simulink model "rectificador_pwm_plecs"  (R2024a)
settings: Solver=ode45  StartTime=0.0  StopTime=10  FixedStep=sim_sample_time  MaxStep=0.0001  RelTol=1e-3
undefined symbols (not defined in the file or in its folder): config, plecs
libraries: slpidlib x3
settings Model: SimulationMode=accelerator  PauseTimes=0.05  Creator=sebar  LastModifiedBy=sebar
settings SolverCC: AlgebraicLoopSolver=TrustRegion  AutoInsertRateTranBlk=on  DecoupledContinuousIntegration=on  ODENIntegrationMethod=ode14x
settings DataIOCC: ExternalInput=getinputstruct(op_trim1)  InitialState=steady_state  LimitDataPoints=on  SaveFinalState=on  SaveFormat=Structure  SaveOutput=off  SignalLogging=off  DSMLogging=off  SaveTime=off
settings OptimizationCC: LifeSpan=inf
settings DebuggingCC: ReadBeforeWriteMsg=DisableAll  WriteAfterWriteMsg=DisableAll  WriteAfterReadMsg=DisableAll  IgnoredZcDiagnostic=none  SolverPrmCheckMsg=warning  MultiTaskDSMMsg=none  SFUnexpectedBacktrackingDiag=warning  SFNoUnconditionalDefaultTransitionDiag=warning  SFExecutionAtInitializationDiag=none  ArithmeticOperatorsInVariantConditions=warning
settings HardwareCC: ProdBitPerPointer=32  ProdBitPerSizeT=32  ProdBitPerPtrDiffT=32  ProdLargestAtomicFloat=None  ProdIntDivRoundTo=Undefined  ProdEndianess=Unspecified  ProdWordSize=32  ProdHWDeviceType=32-bit Generic
settings ModelReferenceCC: UpdateModelReferenceTargets=IfOutOfDate  PropagateSignalLabelsOutOfModel=off
settings SFSimCC: SFSimEcho=off  SimUseLocalCustomCode=off  CustomCodeUndefinedFunction=UseInterfaceOnly  SimTargetLang=C++  GPUAcceleration=on  SimDLTargetLibrary=cudnn
settings RTWCC: RTWUseLocalCustomCode=off  GPUComputeCapability=3.5
settings CodeAppCC: StateflowObjectComments=on
settings GRTTargetCC: TargetLangStandard=C89/C90 (ANSI)
settings ConfigComp: CovMetricSettings=dw  CovSaveCumulativeToWorkspaceVar=on  CovSaveSingleToWorkspaceVar=on  CovExternalEMLEnable=off  CovSFcnEnable=off
settings SimscapeCC: SimscapeNormalizeSystem=off

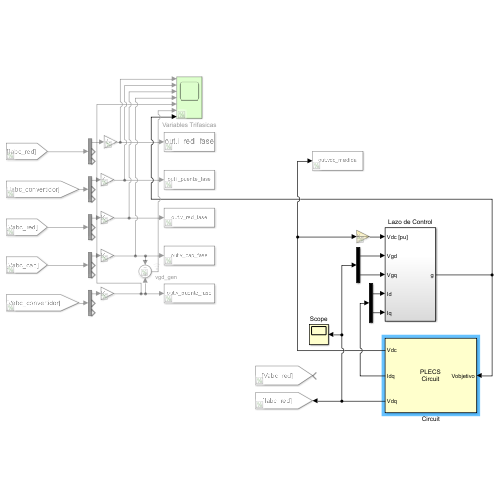
[thumbnail: Simulink's stored preview of the top-level diagram]
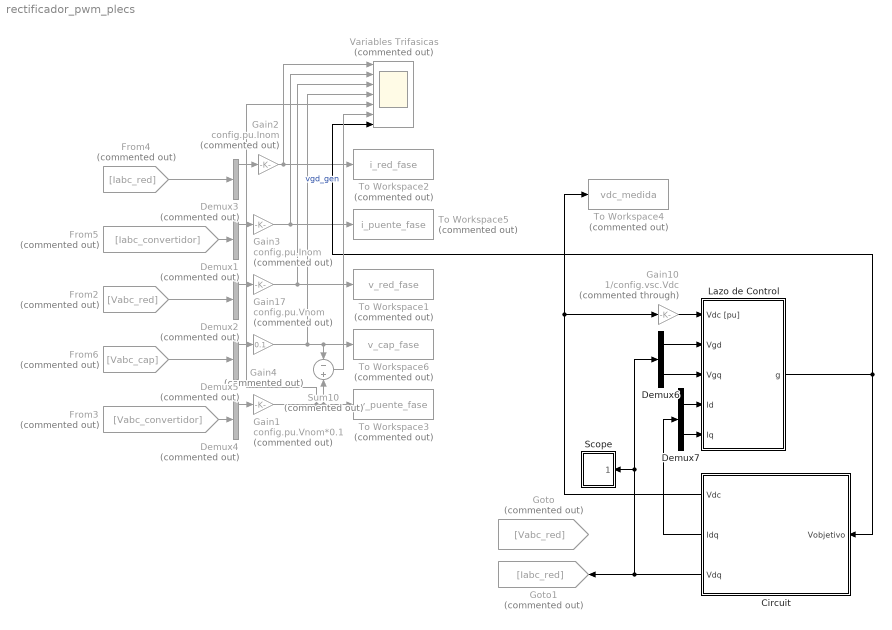
== system rectificador_pwm_plecs ==
  Circuit : Subsystem  LoadFcn=plecs('sl', 200);  InitFcn=plecs('sl', 214);  StartFcn=plecs('sl', 208);  StopFcn=plecs('sl', 209);  mask(PlecsCircuit){PLECSData=<binary blob, 10204 chars, not shown>}
      mask prompts: PLECSData "PLECS Data (Do not delete or modify!)"
      mask init:
      | % PLACE CUSTOM INITIALIZATIONS ABOVE
      | % DO NOT REMOVE
      | plecs('sl', 215);
      | % DO NOT REMOVE
      settings: CopyFcn=plecs('sl', 203);  DeleteFcn=plecs('sl', 205);  UndoDeleteFcn=plecs('sl', 206);  PreSaveFcn=plecs('sl', 211);  PostSaveFcn=plecs('sl', 201);  NameChangeFcn=plecs('sl', 210);  DestroyFcn=plecs('sl', 207);  PreCopyFcn=plecs('sl', 216);  OpenFcn=plecs('sl', 202);  ErrorFcn=plerrorfcn
      mask Help: eval('plecs(''help'', ''qthelp:///creatingacircuit.html'')')
      mask Display: disp('PLECS\nCircuit')
  Demux{1..5} (5 alike) : Demux  Commented=on  Outputs=3
  Demux6 : Demux  Outputs=2
  Demux7 : Demux  Outputs=2
  From2 : From  Commented=on  GotoTag=Vabc_red
  From3 : From  Commented=on  GotoTag=Vabc_convertidor
  From4 : From  Commented=on  GotoTag=Iabc_red
  From5 : From  Commented=on  GotoTag=Iabc_convertidor
  From6 : From  Commented=on  GotoTag=Vabc_cap
  Gain1 : Gain  Commented=on  Gain=config.pu.Vnom*0.1
  Gain10 : Gain  Commented=through  Gain=1/config.vsc.Vdc
  Gain17 : Gain  Commented=on  Gain=config.pu.Vnom
  Gain2 : Gain  Commented=on  Gain=config.pu.Inom
  Gain3 : Gain  Commented=on  Gain=config.pu.Inom
  Gain4 : Gain  Commented=on  Gain=0.1
  Goto : Goto  Commented=on  GotoTag=Vabc_red
  Goto1 : Goto  Commented=on  GotoTag=Iabc_red
  Lazo de Control : Subsystem
  Scope : Subsystem  LoadFcn=plecs('sl', 300);  InitFcn=plecs('sl', 314);  StartFcn=plecs('sl', 308);  StopFcn=plecs('sl', 309);  mask{Settings=<binary blob, 728 chars, not shown>}
      mask init:
      | plecs('sl', 315);
      settings: CopyFcn=plecs('sl', 303);  DeleteFcn=plecs('sl', 305);  UndoDeleteFcn=plecs('sl', 306);  PreSaveFcn=plecs('sl', 311);  NameChangeFcn=plecs('sl', 310);  DestroyFcn=plecs('sl', 307);  OpenFcn=plecs('sl', 302);  ErrorFcn=plerrorfcn
      mask Display: plot([0.1 0.9 0.9 0.1 0.1], [0.9 0.9 0.5 0.5 0.9])
  Sum10 : Sum  Commented=on  Inputs=-|+
  To Workspace1 : ToWorkspace  Commented=on  VariableName=v_red_fase  SaveFormat=Timeseries  SampleTime=config.to_workspace_sample_time
  To Workspace2 : ToWorkspace  Commented=on  VariableName=i_red_fase  SaveFormat=Timeseries  SampleTime=config.to_workspace_sample_time
  To Workspace3 : ToWorkspace  Commented=on  VariableName=v_puente_fase  SaveFormat=Timeseries  SampleTime=config.to_workspace_sample_time
  To Workspace4 : ToWorkspace  Commented=on  VariableName=vdc_medida  SaveFormat=Timeseries  SampleTime=config.to_workspace_sample_time
  To Workspace5 : ToWorkspace  Commented=on  VariableName=i_puente_fase  SaveFormat=Timeseries  SampleTime=config.to_workspace_sample_time
  To Workspace6 : ToWorkspace  Commented=on  VariableName=v_cap_fase  SaveFormat=Timeseries  SampleTime=config.to_workspace_sample_time
  Variables Trifasicas : Scope  Commented=on  NumInputPorts=7
  wires:
  Gain10/1 -> Lazo de Control/1(Vdc [pu])
  Circuit/1(Vdc) -> To Workspace4/1, Gain10/1
  Gain17/1 -> To Workspace1/1, Variables Trifasicas/3
  Gain1/1 -> Sum10/2, To Workspace3/1, Variables Trifasicas/5
  Gain2/1 -> Variables Trifasicas/1, To Workspace2/1
  Gain3/1 -> Variables Trifasicas/2, To Workspace5/1
  Lazo de Control/1(g) -> Circuit/1(Vobjetivo), Variables Trifasicas/7
  From4/1 -> Demux3/1
  Demux3/1 -> Gain2/1
  Demux1/1 -> Gain3/1
  Demux2/1 -> Gain17/1
  Demux4/1 -> Gain1/1
  From3/1 -> Demux4/1
  From2/1 -> Demux2/1
  From5/1 -> Demux1/1
  From6/1 -> Demux5/1
  Gain4/1 -> Sum10/1, To Workspace6/1, Variables Trifasicas/4
  Demux5/1 -> Gain4/1
  Sum10/1 -> Variables Trifasicas/6  "vgd_gen"
  Circuit/3(Vdq) -> Goto1/1, Demux6/1, Scope/1(1)
  Demux6/1 -> Lazo de Control/2(Vgd)
  Demux6/2 -> Lazo de Control/3(Vgq)
  Circuit/2(Idq) -> Demux7/1
  Demux7/1 -> Lazo de Control/4(Id)
  Demux7/2 -> Lazo de Control/5(Iq)

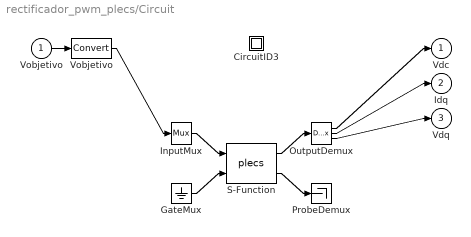
== system rectificador_pwm_plecs/Circuit ==
  Vobjetivo : Inport  PortDimensions=2
  " CircuitID3 " : Subsystem
  " GateMux " : Ground
  " InputMux " : Mux  Inputs=[ 2 ]
  " OutputDemux " : Demux  Outputs=[ 1 2 2 ]
  " ProbeDemux " : Terminator
  " S-Function " : S-Function  FunctionName=plecs  SFunctionDeploymentMode=off  EnableBusSupport=off
  " Vobjetivo " : DataTypeConversion
  Vdc : Outport  PortDimensions=1
  Idq : Outport  Port=2  PortDimensions=2
  Vdq : Outport  Port=3  PortDimensions=2
  wires:
  " InputMux "/1 -> " S-Function "/1
  " GateMux "/1 -> " S-Function "/2
  " S-Function "/1 -> " OutputDemux "/1
  " S-Function "/2 -> " ProbeDemux "/1
  Vobjetivo/1 -> " Vobjetivo "/1
  " Vobjetivo "/1 -> " InputMux "/1
  " OutputDemux "/1 -> Vdc/1
  " OutputDemux "/2 -> Idq/1
  " OutputDemux "/3 -> Vdq/1

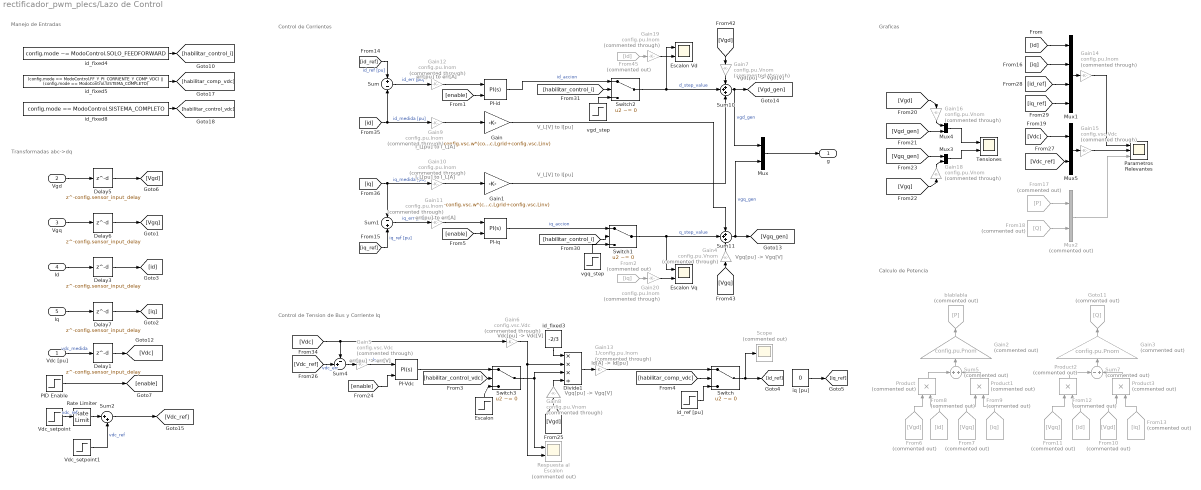
== system rectificador_pwm_plecs/Lazo de Control ==
  note: Transformadas abc->dq
  note: I_L[pu] to I_L[A]
  note: Calculo de Potencia
  note: Graficas
  note: Manejo de Entradas
  note: Control de Tension de Bus y Corriente Iq
  note: Control de Corrientes
  note: V_L[V] to I[pu]
  note: Vgd[pu] -> Vgd[V]
  note: I_L[pu] to I_L[A]
  note: Vgq[pu] -> Vgq[V]
  note: Vgq[pu] -> Vgq[V]
  note: Id[A] -> Id[pu]
  note: err[pu] -> err[V]
  note: err[pu] to err[A]
  note: err[pu] to err[A]
  note: Vdc[pu] -> Vdc[V]
  note: V_L[V] to I[pu]
  Vdc [pu] : Inport
  Vgd : Inport  Port=2
  Vgq : Inport  Port=3
  Id : Inport  Port=4
  Iq : Inport  Port=5
  Delay{1,3,5..7} (5 alike) : Delay  DelayLength=config.sensor_input_delay  InitialCondition=1  SampleTime=config.sensor_input_sample_time
  Divide1 : Product  Inputs=***/
  Escalon : Step  Time=config.step.id.time  Before=config.step.id.start_value  After=config.step.id.end_value  SampleTime=1e-5
  Escalon Vd : Scope  NumInputPorts=2
  Escalon Vq : Scope  NumInputPorts=2
  From10 : From  Commented=on  GotoTag=Vgd
  From11 : From  Commented=on  GotoTag=Vgq
  From12 : From  Commented=on  GotoTag=id
  From13 : From  Commented=on  GotoTag=iq
  From17 : From  Commented=on  GotoTag=P
  From18 : From  Commented=on  GotoTag=Q
  From2 : From  Commented=on  GotoTag=iq
  From45 : From  Commented=on  GotoTag=id
  From6 : From  Commented=on  GotoTag=Vgd
  From7 : From  Commented=on  GotoTag=Vgq
  From8 : From  Commented=on  GotoTag=id
  From9 : From  Commented=on  GotoTag=iq
  Gain : Gain  Gain=config.vsc.w*(config.vsc.Lgrid+config.vsc.Linv)
  Gain1 : Gain  Gain=-config.vsc.w*(config.vsc.Lgrid+config.vsc.Linv)
  Gain{9..12,14,19..20} (7 alike) : Gain  Commented=through  Gain=config.pu.Inom
  Gain13 : Gain  Commented=through  Gain=1/config.pu.Inom
  Gain15 : Gain  Commented=through  Gain=config.vsc.Vdc
  Gain{4,7..8,16,18} (5 alike) : Gain  Commented=through  Gain=config.pu.Vnom
  Gain2 : Gain  Commented=on  Gain=config.pu.Pnom
  Gain3 : Gain  Commented=on  Gain=config.pu.Pnom
  Gain5 : Gain  Commented=through  Gain=config.vsc.Vdc
  Gain6 : Gain  Commented=through  Gain=config.vsc.Vdc
  Goto11 : Goto  Commented=on  GotoTag=Q
  Mux{,3..5} (4 alike) : Mux  Inputs=2
  Mux1 : Mux
  Mux2 : Mux  Commented=on  Inputs=2
  PI-Vdc : slpidlib/PID Controller  Controller=PI  Form=Parallel  TimeDomain=Continuous-time  UseExternalTs=off  SampleTime=1  IntegratorMethod=Forward Euler  FilterMethod=Forward Euler  ControllerParametersSource=internal  P=config.ContDC.Kp  I=config.ContDC.Ki  UseKiTs=off  D=0  UseExternalDerivativeSource=off  N=100  UseFilter=on  TunerSelectOption=Transfer Function Based (PID Tuner App)  InitialConditionSource=internal  InitialConditionForIntegrator=12.92  InitialConditionForFilter=0  DifferentiatorICPrevScaledInput=0  ExternalReset=level  TrackingMode=off  Kt=1  LimitOutput=off  SatLimitsSource=internal  UpperSaturationLimit=inf  LowerSaturationLimit=-inf  LinearizeAsGain=on  AntiWindupMode=none  Kb=1  LimitIntegrator=off  UpperIntegratorSaturationLimit=inf  LowerIntegratorSaturationLimit=-inf  POutMin=[]  POutMax=[]  IOutMin=[]  IOutMax=[]  DOutMin=[]  DOutMax=[]  NOutMin=[]  NOutMax=[]  SumOutMin=[]  SumOutMax=[]  SaturationOutMin=[]  SaturationOutMax=[]  PParamMin=[]  PParamMax=[]  IParamMin=[]  IParamMax=[]  DParamMin=[]  DParamMax=[]  NParamMin=[]  NParamMax=[]  KbParamMin=[]  KbParamMax=[]  KtParamMin=[]  KtParamMax=[]  KbOutMin=[]  KbOutMax=[]  KtOutMin=[]  KtOutMax=[]  IntegratorOutMin=[]  IntegratorOutMax=[]  FilterOutMin=[]  FilterOutMax=[]  SumI1OutMin=[]  SumI1OutMax=[]  SumI2OutMin=[]  SumI2OutMax=[]  SumI3OutMin=[]  SumI3OutMax=[]  SumI4OutMin=[]  SumI4OutMax=[]  SumDOutMin=[]  SumDOutMax=[]  DifferentiatorOutMin=[]  DifferentiatorOutMax=[]  FilterDiffOutCoefMin=[]  FilterDiffOutCoefMax=[]  ReciprocalOutMin=[]  ReciprocalOutMax=[]  SumDenOutMin=[]  SumDenOutMax=[]  SumNumOutMin=[]  SumNumOutMax=[]  DivideOutMin=[]  DivideOutMax=[]  UdiffTsProdOutMin=[]  UdiffTsProdOutMax=[]  NTsProdOutMin=[]  NTsProdOutMax=[]  UintegralTsProdOutMin=[]  UintegralTsProdOutMax=[]  UngainTsProdOutMin=[]  UngainTsProdOutMax=[]  ClampingZeroOutDataTypeStr=Inherit: Inherit via back propagation  ClampingZeroOutMin=[]  ClampingZeroOutMax=[]  FilterDenConstantOutDataTypeStr=Inherit: Inherit via back propagation  FilterDenConstantOutMin=[]  FilterDenConstantOutMax=[]  PCopyOutDataTypeStr=Inherit: Inherit via back propagation  PCopyOutMin=[]  PCopyOutMax=[]  NCopyOutDataTypeStr=Inherit: Inherit via back propagation  NCopyOutMin=[]  NCopyOutMax=[]  IntegratorContinuousStateAttributes=''  IntegratorStateMustResolveToSignalObject=off  IntegratorRTWStateStorageClass=Auto  FilterContinuousStateAttributes=''  FilterStateMustResolveToSignalObject=off  FilterRTWStateStorageClass=Auto  ParallelPVariant=InternalParameters  IdealPVariant=Disabled  IVariant=InternalParameters  DVariant=Disabled  IntegratorVariant=Continuous  SatVariant=Disabled  AWVariant=Passthrough  PCopyVariant=Disabled  TRVariant=Disabled  FdbkBlocksVariant=Forward  IdealPFdbkVariant=Disabled  SatFdbkVariant=Disabled  DerivativeFilterVariant=Disabled  NVariant=Disabled  NCopyVariant=Disabled_SignalSpec  FilterICVariant=Disabled  IntegratorICVariant=InternalICs  ExternalResetVariant=ExternalReset  TRSumVariant=Passthrough  SumFdbkVariant=Disabled  SumVariant=Sum_PI  TsampFilterVariant=InternalTs  TsampNgainVariant=Passthrough  TsampIntegralVariant=Disabled_SignalSpec  ExternalSaturationOutDataTypeStr=Inherit: Same as second input  DerivativeSourceVariant=Disabled
  PI-id : slpidlib/PID Controller  Controller=PI  Form=Parallel  TimeDomain=Continuous-time  UseExternalTs=off  SampleTime=1  IntegratorMethod=Forward Euler  FilterMethod=Forward Euler  ControllerParametersSource=internal  P=config.ContI.Kp  I=config.ContI.Ki  UseKiTs=off  D=0  UseExternalDerivativeSource=off  N=100  UseFilter=on  TunerSelectOption=Transfer Function Based (PID Tuner App)  InitialConditionSource=internal  InitialConditionForIntegrator=-1.85  InitialConditionForFilter=0  DifferentiatorICPrevScaledInput=0  ExternalReset=level  TrackingMode=off  Kt=1  LimitOutput=off  SatLimitsSource=internal  UpperSaturationLimit=-4  LowerSaturationLimit=-20  LinearizeAsGain=on  AntiWindupMode=clamping  Kb=1  LimitIntegrator=off  UpperIntegratorSaturationLimit=inf  LowerIntegratorSaturationLimit=-inf  POutMin=[]  POutMax=[]  IOutMin=[]  IOutMax=[]  DOutMin=[]  DOutMax=[]  NOutMin=[]  NOutMax=[]  SumOutMin=[]  SumOutMax=[]  SaturationOutMin=[]  SaturationOutMax=[]  PParamMin=[]  PParamMax=[]  IParamMin=[]  IParamMax=[]  DParamMin=[]  DParamMax=[]  NParamMin=[]  NParamMax=[]  KbParamMin=[]  KbParamMax=[]  KtParamMin=[]  KtParamMax=[]  KbOutMin=[]  KbOutMax=[]  KtOutMin=[]  KtOutMax=[]  IntegratorOutMin=[]  IntegratorOutMax=[]  FilterOutMin=[]  FilterOutMax=[]  SumI1OutMin=[]  SumI1OutMax=[]  SumI2OutMin=[]  SumI2OutMax=[]  SumI3OutMin=[]  SumI3OutMax=[]  SumI4OutMin=[]  SumI4OutMax=[]  SumDOutMin=[]  SumDOutMax=[]  DifferentiatorOutMin=[]  DifferentiatorOutMax=[]  FilterDiffOutCoefMin=[]  FilterDiffOutCoefMax=[]  ReciprocalOutMin=[]  ReciprocalOutMax=[]  SumDenOutMin=[]  SumDenOutMax=[]  SumNumOutMin=[]  SumNumOutMax=[]  DivideOutMin=[]  DivideOutMax=[]  UdiffTsProdOutMin=[]  UdiffTsProdOutMax=[]  NTsProdOutMin=[]  NTsProdOutMax=[]  UintegralTsProdOutMin=[]  UintegralTsProdOutMax=[]  UngainTsProdOutMin=[]  UngainTsProdOutMax=[]  ClampingZeroOutDataTypeStr=Inherit: Inherit via back propagation  ClampingZeroOutMin=[]  ClampingZeroOutMax=[]  FilterDenConstantOutDataTypeStr=Inherit: Inherit via back propagation  FilterDenConstantOutMin=[]  FilterDenConstantOutMax=[]  PCopyOutDataTypeStr=Inherit: Inherit via back propagation  PCopyOutMin=[]  PCopyOutMax=[]  NCopyOutDataTypeStr=Inherit: Inherit via back propagation  NCopyOutMin=[]  NCopyOutMax=[]  IntegratorContinuousStateAttributes=''  IntegratorStateMustResolveToSignalObject=off  IntegratorRTWStateStorageClass=Auto  FilterContinuousStateAttributes=''  FilterStateMustResolveToSignalObject=off  FilterRTWStateStorageClass=Auto  ParallelPVariant=InternalParameters  IdealPVariant=Disabled  IVariant=InternalParameters  DVariant=Disabled  IntegratorVariant=Continuous  SatVariant=Disabled  AWVariant=Passthrough  PCopyVariant=Disabled  TRVariant=Disabled  FdbkBlocksVariant=Forward  IdealPFdbkVariant=Disabled  SatFdbkVariant=Disabled  DerivativeFilterVariant=Disabled  NVariant=Disabled  NCopyVariant=Disabled_SignalSpec  FilterICVariant=Disabled  IntegratorICVariant=InternalICs  ExternalResetVariant=ExternalReset  TRSumVariant=Passthrough  SumFdbkVariant=Disabled  SumVariant=Sum_PI  TsampFilterVariant=InternalTs  TsampNgainVariant=Passthrough  TsampIntegralVariant=Disabled_SignalSpec  ExternalSaturationOutDataTypeStr=Inherit: Same as second input  DerivativeSourceVariant=Disabled
  PI-iq : slpidlib/PID Controller  Controller=PI  Form=Parallel  TimeDomain=Continuous-time  UseExternalTs=off  SampleTime=1  IntegratorMethod=Forward Euler  FilterMethod=Forward Euler  ControllerParametersSource=internal  P=config.ContI.Kp  I=config.ContI.Ki  UseKiTs=off  D=0  UseExternalDerivativeSource=off  N=100  UseFilter=on  TunerSelectOption=Transfer Function Based (PID Tuner App)  InitialConditionSource=internal  InitialConditionForIntegrator=0  InitialConditionForFilter=0  DifferentiatorICPrevScaledInput=0  ExternalReset=level  TrackingMode=off  Kt=1  LimitOutput=off  SatLimitsSource=internal  UpperSaturationLimit=20  LowerSaturationLimit=-20  LinearizeAsGain=on  AntiWindupMode=none  Kb=1  LimitIntegrator=off  UpperIntegratorSaturationLimit=inf  LowerIntegratorSaturationLimit=-inf  POutMin=[]  POutMax=[]  IOutMin=[]  IOutMax=[]  DOutMin=[]  DOutMax=[]  NOutMin=[]  NOutMax=[]  SumOutMin=[]  SumOutMax=[]  SaturationOutMin=[]  SaturationOutMax=[]  PParamMin=[]  PParamMax=[]  IParamMin=[]  IParamMax=[]  DParamMin=[]  DParamMax=[]  NParamMin=[]  NParamMax=[]  KbParamMin=[]  KbParamMax=[]  KtParamMin=[]  KtParamMax=[]  KbOutMin=[]  KbOutMax=[]  KtOutMin=[]  KtOutMax=[]  IntegratorOutMin=[]  IntegratorOutMax=[]  FilterOutMin=[]  FilterOutMax=[]  SumI1OutMin=[]  SumI1OutMax=[]  SumI2OutMin=[]  SumI2OutMax=[]  SumI3OutMin=[]  SumI3OutMax=[]  SumI4OutMin=[]  SumI4OutMax=[]  SumDOutMin=[]  SumDOutMax=[]  DifferentiatorOutMin=[]  DifferentiatorOutMax=[]  FilterDiffOutCoefMin=[]  FilterDiffOutCoefMax=[]  ReciprocalOutMin=[]  ReciprocalOutMax=[]  SumDenOutMin=[]  SumDenOutMax=[]  SumNumOutMin=[]  SumNumOutMax=[]  DivideOutMin=[]  DivideOutMax=[]  UdiffTsProdOutMin=[]  UdiffTsProdOutMax=[]  NTsProdOutMin=[]  NTsProdOutMax=[]  UintegralTsProdOutMin=[]  UintegralTsProdOutMax=[]  UngainTsProdOutMin=[]  UngainTsProdOutMax=[]  ClampingZeroOutDataTypeStr=Inherit: Inherit via back propagation  ClampingZeroOutMin=[]  ClampingZeroOutMax=[]  FilterDenConstantOutDataTypeStr=Inherit: Inherit via back propagation  FilterDenConstantOutMin=[]  FilterDenConstantOutMax=[]  PCopyOutDataTypeStr=Inherit: Inherit via back propagation  PCopyOutMin=[]  PCopyOutMax=[]  NCopyOutDataTypeStr=Inherit: Inherit via back propagation  NCopyOutMin=[]  NCopyOutMax=[]  IntegratorContinuousStateAttributes=''  IntegratorStateMustResolveToSignalObject=off  IntegratorRTWStateStorageClass=Auto  FilterContinuousStateAttributes=''  FilterStateMustResolveToSignalObject=off  FilterRTWStateStorageClass=Auto  ParallelPVariant=InternalParameters  IdealPVariant=Disabled  IVariant=InternalParameters  DVariant=Disabled  IntegratorVariant=Continuous  SatVariant=Disabled  AWVariant=Passthrough  PCopyVariant=Disabled  TRVariant=Disabled  FdbkBlocksVariant=Forward  IdealPFdbkVariant=Disabled  SatFdbkVariant=Disabled  DerivativeFilterVariant=Disabled  NVariant=Disabled  NCopyVariant=Disabled_SignalSpec  FilterICVariant=Disabled  IntegratorICVariant=InternalICs  ExternalResetVariant=ExternalReset  TRSumVariant=Passthrough  SumFdbkVariant=Disabled  SumVariant=Sum_PI  TsampFilterVariant=InternalTs  TsampNgainVariant=Passthrough  TsampIntegralVariant=Disabled_SignalSpec  ExternalSaturationOutDataTypeStr=Inherit: Same as second input  DerivativeSourceVariant=Disabled
  PID Enable : Step  Time=1.5  Before=1  After=0  SampleTime=1e-5
  Parametros Relevantes : Scope  NumInputPorts=3
  Product{,1..3} (4 alike) : Product  Commented=on
  Rate Limiter : RateLimiter  RisingSlewLimit=15  SampleTimeMode=inherited
  Respuesta al Escalon : Scope  Commented=on  NumInputPorts=2
  Scope : Scope  Commented=on
  Sum : Sum  Inputs=+|-
  Sum1 : Sum  Inputs=-|+
  Sum10 : Sum  Inputs=+++
  Sum11 : Sum  Inputs=+++
  Sum2 : Sum  Inputs=|++
  Sum4 : Sum  Inputs=-+|
  Sum5 : Sum  Commented=on  Inputs=+|+
  Sum7 : Sum  Commented=on  Inputs=-|+
  Switch{,1..3} (4 alike) : Switch  Criteria=u2 ~= 0  SaturateOnIntegerOverflow=off  InputSameDT=off
  Tensiones : Scope  NumInputPorts=2
  Vdc_setpoint : Step  Time=1.5  Before=config.vsc.Vgrid*sqrt(2)*3*sqrt(3)/pi*0+350  After=config.vsc.Vdc*0+350  SampleTime=0
  Vdc_setpoint1 : Step  Time=7  After=50  SampleTime=0
  blablabla : Goto  Commented=on  GotoTag=P
  id_fixed3 : Constant  Value=-2/3
  id_fixed4 : Constant  Value=config.mode ~= ModoControl.SOLO_FEEDFORWARD
  id_fixed5 : Constant  Value=(config.mode == ModoControl.FF_Y_PI_CORRIENTE_Y_COMP_VDC) || (config.mode == ModoControl.SISTEMA_COMPLETO)
  id_fixed8 : Constant  Value=config.mode == ModoControl.SISTEMA_COMPLETO
  id_ref [pu] : Step  Time=1.25  Before=-3.0707/config.pu.Inom  After=-3.0707/config.pu.Inom*(1 + config.step_setpoint_corriente/100)  SampleTime=0
  iq [pu] : Constant  Value=0
  vgd_step : Step  Time=config.step.vgd.time  Before=config.step.vgd.start_value  After=config.step.vgd.end_value  SampleTime=1e-5
  vgq_step : Step  Time=config.step.vgq.time  Before=config.step.vgq.start_value  After=config.step.vgq.end_value  SampleTime=1e-5
  g : Outport
  wires:
  Vgq/1 -> Delay6/1
  [id] -> Gain9/1, Sum/2  "id_medida [pu]"
  [iq] -> Gain10/1, Sum1/1  "iq_medida [pu]"
  [id_ref] -> Sum/1  "id_ref [pu]"
  [iq_ref] -> Sum1/2  "iq_ref [pu]"
  Sum/1 -> Gain12/1  "id_err [pu]"
  Sum1/1 -> Gain11/1  "iq_err [pu]"
  PI-iq/1 -> Switch1/1  "iq_accion"
  Sum11/1 -> Mux/2, [Vgq_gen]  "vgq_gen"
  Vdc [pu]/1 -> Delay1/1  "vdc_medida"
  Gain5/1 -> PI-Vdc/1  "vdc_err"
  Divide1/1 -> Gain13/1
  id_ref [pu]/1 -> Switch/3
  iq [pu]/1 -> [iq_ref]
  From17/1 -> Mux2/1
  From18/1 -> Mux2/2
  [iq] -> Mux1/2
  [id] -> Mux1/1
  [Vdc] -> Mux5/1
  Mux1/1 -> Gain14/1
  Mux2/1 -> Parametros Relevantes/3
  [Vgd_gen] -> Mux4/2
  [Vgq_gen] -> Mux3/1
  Switch3/1 -> Divide1/3, Respuesta al Escalon/1
  [Vgd] -> Gain8/1
  Mux5/1 -> Gain15/1
  [Vdc_ref] -> Mux5/2
  [id_ref] -> Mux1/3
  [iq_ref] -> Mux1/4
  [habilitar_control_i] -> Switch1/2
  [habilitar_control_i] -> Switch2/2
  PI-id/1 -> Switch2/1  "id_accion"
  [Vdc] -> Gain6/1, Sum4/1
  Sum10/1 -> Mux/1, [Vgd_gen]  "vgd_gen"
  vgd_step/1 -> Switch2/3
  vgq_step/1 -> Switch1/3
  Switch2/1 -> Sum10/2, Escalon Vd/1  "d_step_value"
  [Vgd] -> Gain7/1
  Switch1/1 -> Sum11/2, Escalon Vq/1  "q_step_value"
  id_fixed3/1 -> Divide1/1
  From45/1 -> Gain19/1
  PI-Vdc/1 -> Switch3/1
  [habilitar_control_vdc] -> Switch3/2
  Escalon/1 -> Switch3/3
  From7/1 -> Product1/1
  From10/1 -> Product3/1
  From12/1 -> Product2/2
  Product1/1 -> Sum5/2
  Sum5/1 -> Gain2/1
  Sum7/1 -> Gain3/1
  Gain3/1 -> Goto11/1
  From8/1 -> Product/2
  From6/1 -> Product/1
  Product3/1 -> Sum7/2
  Product/1 -> Sum5/1
  From13/1 -> Product3/2
  From11/1 -> Product2/1
  Gain2/1 -> blablabla/1
  From9/1 -> Product1/2
  Product2/1 -> Sum7/1
  Vdc_setpoint/1 -> Rate Limiter/1  "vdc_ref"
  From2/1 -> Gain20/1
  Gain/1 -> Sum11/1
  Gain1/1 -> Sum10/3
  Gain8/1 -> Divide1/4
  Gain10/1 -> Gain1/1
  Gain9/1 -> Gain/1
  Gain7/1 -> Sum10/1
  [Vgq] -> Gain4/1
  Gain4/1 -> Sum11/3
  Gain13/1 -> Switch/1
  Sum4/1 -> Gain5/1
  Gain14/1 -> Parametros Relevantes/1
  Gain15/1 -> Parametros Relevantes/2
  [Vgd] -> Gain16/1
  [Vgq] -> Gain18/1
  Mux4/1 -> Tensiones/1
  Mux3/1 -> Tensiones/2
  Gain16/1 -> Mux4/1
  Gain18/1 -> Mux3/2
  Gain19/1 -> Escalon Vd/2
  Gain20/1 -> Escalon Vq/2
  Delay1/1 -> [Vdc]
  Gain6/1 -> Divide1/2, Respuesta al Escalon/2
  id_fixed4/1 -> [habilitar_control_i]
  [habilitar_comp_vdc] -> Switch/2
  Switch/1 -> [id_ref], Scope/1
  id_fixed5/1 -> [habilitar_comp_vdc]
  id_fixed8/1 -> [habilitar_control_vdc]
  Vgd/1 -> Delay5/1
  Delay5/1 -> [Vgd]
  Delay6/1 -> [Vgq]
  Iq/1 -> Delay7/1
  Id/1 -> Delay3/1
  Delay3/1 -> [id]
  Delay7/1 -> [iq]
  Mux/1 -> g/1
  [Vdc_ref] -> Sum4/2  "vdc_err"
  Gain12/1 -> PI-id/1
  PID Enable/1 -> [enable]
  Gain11/1 -> PI-iq/1
  Vdc_setpoint1/1 -> Sum2/2  "vdc_ref"
  Rate Limiter/1 -> Sum2/1
  Sum2/1 -> [Vdc_ref]
  [enable] -> PI-id/2
  [enable] -> PI-iq/2
  [enable] -> PI-Vdc/2

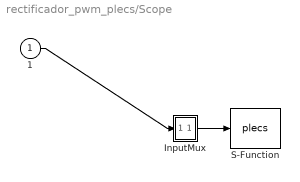
== system rectificador_pwm_plecs/Scope ==
  1 : Inport
  " InputMux " : Subsystem
      mask Display: disp('Mux')
  " S-Function " : S-Function  FunctionName=plecs  SFunctionDeploymentMode=off  EnableBusSupport=off
  wires:
  1/1 -> " InputMux "/1(In1)
  " InputMux "/1(Out) -> " S-Function "/1

== system rectificador_pwm_plecs/Circuit/ CircuitID3  ==

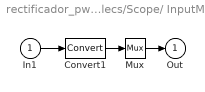
== system rectificador_pwm_plecs/Scope/ InputMux  ==
  In1 : Inport
  Convert1 : DataTypeConversion
  Mux : Mux  Inputs=1
  Out : Outport
  wires:
  Convert1/1 -> Mux/1
  In1/1 -> Convert1/1
  Mux/1 -> Out/1
